simulink model "Pretty_Lin_Hover_Sim"  (R2025b)
settings: Solver=VariableStepAuto  StartTime=0.0  StopTime=10.0  RelTol=1e-3
values from neighbouring files (symbols this model uses):
  A = zeros(12,12)    [lin_hover.m]
  A_kfd = sys_kf_d.A    [lin_hover.m]
  B = zeros(12,4)    [lin_hover.m]
  B_kfd = sys_kf_d.B    [lin_hover.m]
  C11 = 4.58e-4    (= 0.000458)    [lin_hover.m]    (also in non_lin_sim.m)
  g = 9.81    [lin_hover.m]    (also in non_lin_sim.m)
  k_tau = 0.00    (= 0)    [lin_hover.m]    (also in non_lin_sim.m)
  m = 0.110    (= 0.11)    [lin_hover.m]    (also in non_lin_sim.m)
  max_pot = 1950    [lin_hover.m]
  noise_true = 1    [lin_hover.m]
  pitch_D = 0    [lin_hover.m]
  pitch_I = 0.005*Iy/Ix    [lin_hover.m]
  pitch_P = 0.022*Iy/Ix    [lin_hover.m]
  roll_D = 0    [lin_hover.m]
  roll_I = 0.005    [lin_hover.m]
  roll_P = 0.022    [lin_hover.m]
  S = 0.11    [lin_hover.m]    (also in non_lin_sim.m)
  strength = 50    [lin_hover.m]
  tau_wing = 0.1/2.2    (= 0.0454545454545)    [lin_hover.m]
  Ts = 1/fs    (= 0.00025)    [lin_hover.m]
  u0 = (m*g/4 - C21)/C11    (= 1816.10262009)    [lin_hover.m]
  X0 = zeros([12,1])    [lin_hover.m]
  Xref = zeros([12,1])    [lin_hover.m]
  Xu = rho*CDx*Ax*v_ref    (= 0.148971998855)    [lin_hover.m]    (also in non_lin_sim.m)
  yaw_D = 0    [lin_hover.m]
  yaw_I = 0.001    [lin_hover.m]
  yaw_P = 0.001    [lin_hover.m]
  Yv = rho*CDy*Ay*v_ref    (= 0.148971998855)    [lin_hover.m]    (also in non_lin_sim.m)
  Zw = rho*CDz*Az*w_ref    (= 0.104280399198)    [lin_hover.m]    (also in non_lin_sim.m)
undefined symbols (not defined in the file or in its folder): accel, C_kf, D_kf, DiscIntNeverNeededParam, Discrete, gyro, mahoney, R_kf, Time, x_kf0
libraries: slpidlib x5, simulink x3, ctrlSharedLib x1
settings Model: Creator=bmatt  LastModifiedBy=bmatt

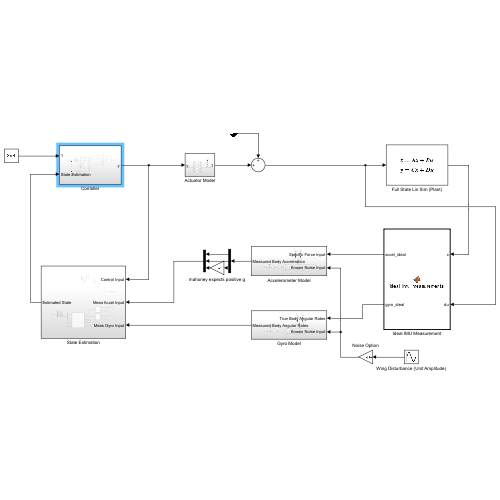
[thumbnail: Simulink's stored preview of the top-level diagram]
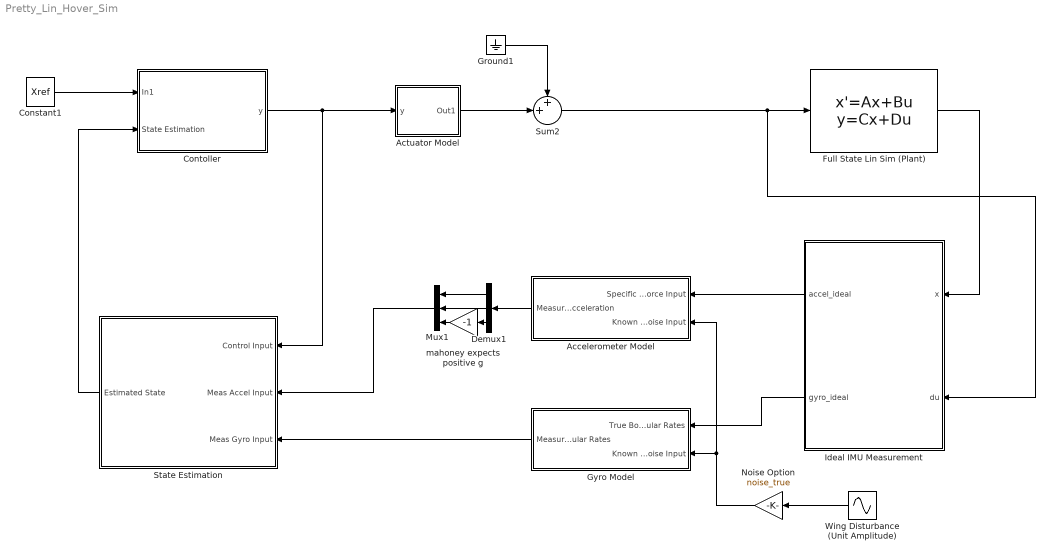
== system Pretty_Lin_Hover_Sim ==
  Accelerometer Model : Subsystem
  Actuator Model : Subsystem
  Constant1 : Constant  Value=Xref  SampleTime=-1
  Contoller : Subsystem
  Demux1 : Demux  Outputs=3
  Full State Lin Sim (Plant) : StateSpace  A=A  B=B  C=eye(12)  D=zeros(12,4)  InitialCondition=X0
  Ground1 : Ground
  Gyro Model : Subsystem
  Ideal IMU Measurement : MATLAB Function  TreatAsAtomicUnit=on
  Mux1 : Mux  Inputs=3
  Noise Option : Gain  Gain=noise_true
  State Estimation : Subsystem
  Sum2 : Sum  Inputs=++|
  Wing Disturbance (Unit Amplitude) : Sin  Frequency=2*pi*24  SampleTime=0
  mahoney expects positive g : Gain  Gain=-1
  wires:
  Sum2/1 -> Ideal IMU Measurement/2(du), Full State Lin Sim (Plant)/1
  Constant1/1 -> Contoller/1(In1)
  Actuator Model/1(Out1) -> Sum2/2
  Noise Option/1 -> Accelerometer Model/2(Known Noise Input), Gyro Model/2(Known Noise Input)
  Mux1/1 -> State Estimation/2(Meas Accel Input)
  Demux1/3 -> mahoney expects positive g/1
  State Estimation/1(Estimated State) -> Contoller/2(State Estimation)
  mahoney expects positive g/1 -> Mux1/3
  Wing Disturbance (Unit Amplitude)/1 -> Noise Option/1
  Ideal IMU Measurement/2(gyro_ideal) -> Gyro Model/1(True Body Angular Rates)
  Gyro Model/1(Measured Body Angular Rates) -> State Estimation/3(Meas Gyro Input)
  Full State Lin Sim (Plant)/1 -> Ideal IMU Measurement/1(x)
  Accelerometer Model/1(Measured Body Acceleration) -> Demux1/1
  Contoller/1(y) -> State Estimation/1(Control Input), Actuator Model/1(y)
  Demux1/1 -> Mux1/1
  Ground1/1 -> Sum2/1
  Demux1/2 -> Mux1/2
  Ideal IMU Measurement/1(accel_ideal) -> Accelerometer Model/1(Specific Force Input)

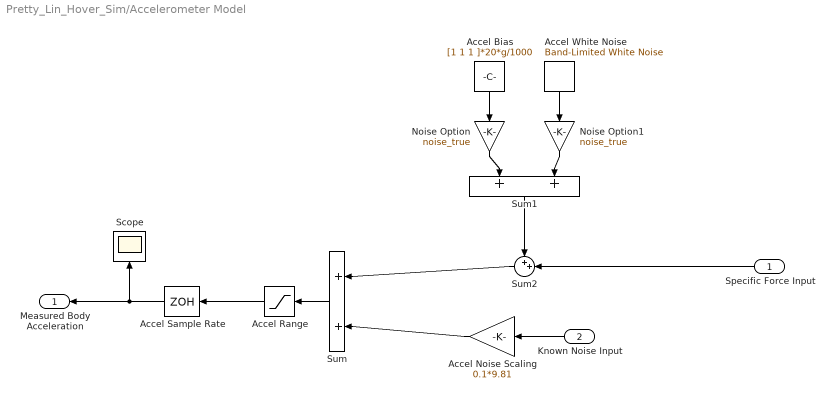
== system Pretty_Lin_Hover_Sim/Accelerometer Model ==
  Specific Force Input : Inport
  Known Noise Input : Inport  Port=2
  Accel White Noise : simulink/Sources/Band-Limited White Noise  Cov=[1 1 1]*((0.16*9.81/1000)*sqrt(740))^2  Ts=1/1600  seed=[23341]
  Accel Bias : Constant  Value=[1 1 1 ]*20*g/1000  SampleTime=1/1600
  Accel Noise Scaling : Gain  Gain=0.1*9.81
  Accel Range : Saturate  UpperLimit=4*9.81  LowerLimit=-4*9.81
  Accel Sample Rate : ZeroOrderHold  SampleTime=1/1600
  Noise Option : Gain  Gain=noise_true
  Noise Option1 : Gain  Gain=noise_true
  Scope : Scope
      settings: ActiveDisplayYMinimum=-1  ActiveDisplayYMaximum=1  DataLoggingVariableName=ScopeData13
  Sum : Sum  Inputs=+|+
  Sum1 : Sum  Inputs=+|+
  Sum2 : Sum  Inputs=++|
  Measured Body Acceleration : Outport
  wires:
  Sum/1 -> Accel Range/1
  Sum2/1 -> Sum/1
  Accel Sample Rate/1 -> Scope/1, Measured Body Acceleration/1
  Known Noise Input/1 -> Accel Noise Scaling/1
  Specific Force Input/1 -> Sum2/2
  Sum1/1 -> Sum2/1
  Accel Noise Scaling/1 -> Sum/2
  Accel Range/1 -> Accel Sample Rate/1
  Noise Option/1 -> Sum1/1
  Accel Bias/1 -> Noise Option/1
  Noise Option1/1 -> Sum1/2
  Accel White Noise/1 -> Noise Option1/1

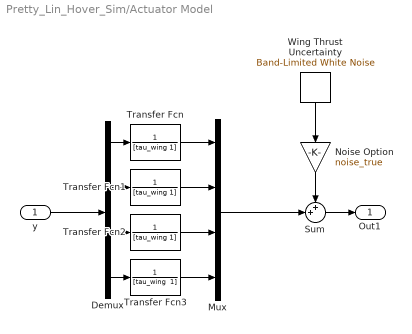
== system Pretty_Lin_Hover_Sim/Actuator Model ==
  y : Inport
  Demux : Demux
  Mux : Mux
  Noise Option : Gain  Gain=noise_true
  Sum : Sum  Inputs=++|
  Transfer Fcn : TransferFcn  Denominator=[tau_wing 1]
  Transfer Fcn1 : TransferFcn  Denominator=[tau_wing 1]
  Transfer Fcn2 : TransferFcn  Denominator=[tau_wing 1]
  Transfer Fcn3 : TransferFcn  Denominator="[tau_wing  1]"
  Wing Thrust Uncertainty : simulink/Sources/Band-Limited White Noise  Cov=1*[0.000001566122567;0.000001566122567;0.000001566122567;0.000001566122567]  Ts=Ts  seed=[23341]
  Out1 : Outport
  wires:
  Demux/4 -> Transfer Fcn3/1
  Demux/1 -> Transfer Fcn/1
  Demux/2 -> Transfer Fcn1/1
  Demux/3 -> Transfer Fcn2/1
  Transfer Fcn/1 -> Mux/1
  Transfer Fcn1/1 -> Mux/2
  Transfer Fcn2/1 -> Mux/3
  Transfer Fcn3/1 -> Mux/4
  y/1 -> Demux/1
  Sum/1 -> Out1/1
  Mux/1 -> Sum/2
  Wing Thrust Uncertainty/1 -> Noise Option/1
  Noise Option/1 -> Sum/1

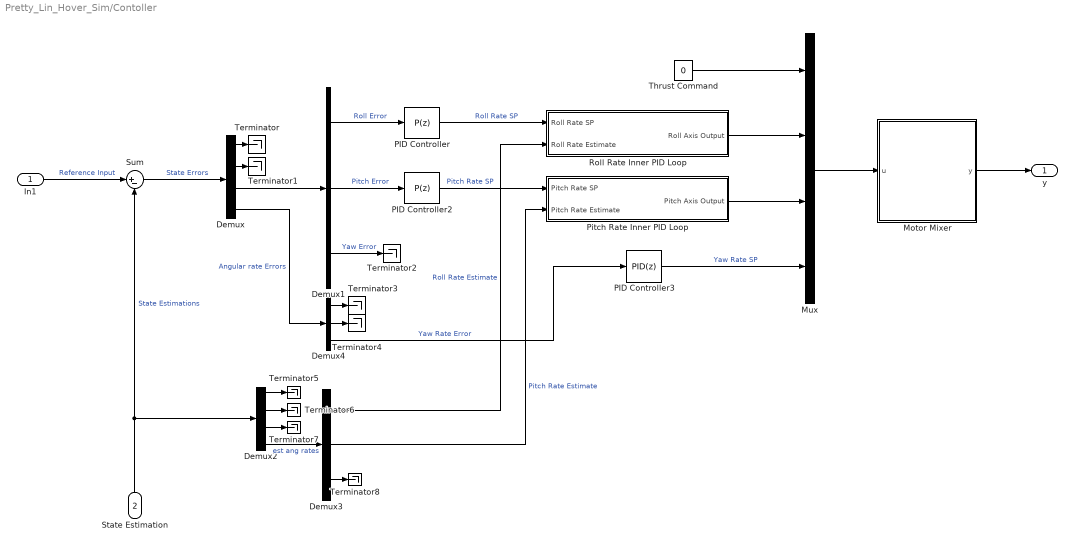
== system Pretty_Lin_Hover_Sim/Contoller ==
  In1 : Inport
  State Estimation : Inport  Port=2
  Demux : Demux  Outputs=[3 3 3 3]
  Demux1 : Demux  Outputs=[1 1 1]
  Demux2 : Demux  Outputs=[3 3 3 3]
  Demux3 : Demux  Outputs=[1 1 1]
  Demux4 : Demux  Outputs=[1 1 1]
  Motor Mixer : Subsystem
  Mux : Mux
  PID Controller : slpidlib/PID Controller  Controller=P  Form=Parallel  TimeDomain=Discrete-time  UseExternalTs=off  SampleTime=Ts  IntegratorMethod=Forward Euler  FilterMethod=Forward Euler  ControllerParametersSource=internal  P=strength/10  I=194.232873086371  UseKiTs=off  D=-0.0894221705749344  UseExternalDerivativeSource=off  N=55.5911819026225  UseFilter=on  TunerSelectOption=Frequency Response Based  InitialConditionSource=internal  InitialConditionForIntegrator=Xref(7) - X0(7)  InitialConditionForFilter=0  DifferentiatorICPrevScaledInput=0  ExternalReset=none  TrackingMode=off  Kt=1  LimitOutput=on  SatLimitsSource=internal  UpperSaturationLimit=3.5  LowerSaturationLimit=-3.5  LinearizeAsGain=on  AntiWindupMode=external  Kb=1  LimitIntegrator=off  UpperIntegratorSaturationLimit=inf  LowerIntegratorSaturationLimit=-inf  POutMin=[]  POutMax=[]  IOutMin=[]  IOutMax=[]  DOutMin=[]  DOutMax=[]  NOutMin=[]  NOutMax=[]  SumOutMin=[]  SumOutMax=[]  SaturationOutMin=[]  SaturationOutMax=[]  PParamMin=[]  PParamMax=[]  IParamMin=[]  IParamMax=[]  DParamMin=[]  DParamMax=[]  NParamMin=[]  NParamMax=[]  KbParamMin=[]  KbParamMax=[]  KtParamMin=[]  KtParamMax=[]  KbOutMin=[]  KbOutMax=[]  KtOutMin=[]  KtOutMax=[]  IntegratorOutMin=[]  IntegratorOutMax=[]  FilterOutMin=[]  FilterOutMax=[]  SumI1OutMin=[]  SumI1OutMax=[]  SumI2OutMin=[]  SumI2OutMax=[]  SumI3OutMin=[]  SumI3OutMax=[]  SumI4OutMin=[]  SumI4OutMax=[]  SumDOutMin=[]  SumDOutMax=[]  DifferentiatorOutMin=[]  DifferentiatorOutMax=[]  FilterDiffOutCoefMin=[]  FilterDiffOutCoefMax=[]  ReciprocalOutMin=[]  ReciprocalOutMax=[]  SumDenOutMin=[]  SumDenOutMax=[]  SumNumOutMin=[]  SumNumOutMax=[]  DivideOutMin=[]  DivideOutMax=[]  UdiffTsProdOutMin=[]  UdiffTsProdOutMax=[]  NTsProdOutMin=[]  NTsProdOutMax=[]  UintegralTsProdOutMin=[]  UintegralTsProdOutMax=[]  UngainTsProdOutMin=[]  UngainTsProdOutMax=[]  ClampingZeroOutDataTypeStr=Inherit: Inherit via back propagation  ClampingZeroOutMin=[]  ClampingZeroOutMax=[]  FilterDenConstantOutDataTypeStr=Inherit: Inherit via back propagation  FilterDenConstantOutMin=[]  FilterDenConstantOutMax=[]  PCopyOutDataTypeStr=Inherit: Inherit via back propagation  PCopyOutMin=[]  PCopyOutMax=[]  NCopyOutDataTypeStr=Inherit: Inherit via back propagation  NCopyOutMin=[]  NCopyOutMax=[]  IntegratorContinuousStateAttributes=''  IntegratorStateMustResolveToSignalObject=off  IntegratorRTWStateStorageClass=Auto  FilterContinuousStateAttributes=''  FilterStateMustResolveToSignalObject=off  FilterRTWStateStorageClass=Auto  ParallelPVariant=InternalParameters  IdealPVariant=Disabled  IVariant=Disabled  DVariant=Disabled  IntegratorVariant=Disabled  SatVariant=Enabled  AWVariant=Disabled  PCopyVariant=Disabled  TRVariant=Disabled  FdbkBlocksVariant=Forward  IdealPFdbkVariant=Disabled  SatFdbkVariant=Disabled  DerivativeFilterVariant=Disabled  NVariant=Disabled  NCopyVariant=Disabled_SignalSpec  FilterICVariant=Disabled  IntegratorICVariant=Disabled  ExternalResetVariant=Disabled  TRSumVariant=Passthrough  SumFdbkVariant=Disabled  SumVariant=Passthrough_P  TsampFilterVariant=InternalTs  TsampNgainVariant=Passthrough  TsampIntegralVariant=Disabled_SignalSpec  ExternalSaturationOutDataTypeStr=Inherit: Same as second input  DerivativeSourceVariant=Disabled  PreIntVariant=InternalPreInt
  PID Controller2 : slpidlib/PID Controller  Controller=P  Form=Parallel  TimeDomain=Discrete-time  UseExternalTs=off  SampleTime=Ts  IntegratorMethod=Forward Euler  FilterMethod=Forward Euler  ControllerParametersSource=internal  P=strength/10  I=0.287608182877056  UseKiTs=off  D=0  UseExternalDerivativeSource=off  N=100  UseFilter=on  TunerSelectOption=Transfer Function Based (PID Tuner App)  InitialConditionSource=internal  InitialConditionForIntegrator=Xref(8) - X0(8)  InitialConditionForFilter=0  DifferentiatorICPrevScaledInput=0  ExternalReset=none  TrackingMode=off  Kt=1  LimitOutput=on  SatLimitsSource=internal  UpperSaturationLimit=3.5  LowerSaturationLimit=-3.5  LinearizeAsGain=off  AntiWindupMode=none  Kb=1  LimitIntegrator=off  UpperIntegratorSaturationLimit=inf  LowerIntegratorSaturationLimit=-inf  POutMin=[]  POutMax=[]  IOutMin=[]  IOutMax=[]  DOutMin=[]  DOutMax=[]  NOutMin=[]  NOutMax=[]  SumOutMin=[]  SumOutMax=[]  SaturationOutMin=[]  SaturationOutMax=[]  PParamMin=[]  PParamMax=[]  IParamMin=[]  IParamMax=[]  DParamMin=[]  DParamMax=[]  NParamMin=[]  NParamMax=[]  KbParamMin=[]  KbParamMax=[]  KtParamMin=[]  KtParamMax=[]  KbOutMin=[]  KbOutMax=[]  KtOutMin=[]  KtOutMax=[]  IntegratorOutMin=[]  IntegratorOutMax=[]  FilterOutMin=[]  FilterOutMax=[]  SumI1OutMin=[]  SumI1OutMax=[]  SumI2OutMin=[]  SumI2OutMax=[]  SumI3OutMin=[]  SumI3OutMax=[]  SumI4OutMin=[]  SumI4OutMax=[]  SumDOutMin=[]  SumDOutMax=[]  DifferentiatorOutMin=[]  DifferentiatorOutMax=[]  FilterDiffOutCoefMin=[]  FilterDiffOutCoefMax=[]  ReciprocalOutMin=[]  ReciprocalOutMax=[]  SumDenOutMin=[]  SumDenOutMax=[]  SumNumOutMin=[]  SumNumOutMax=[]  DivideOutMin=[]  DivideOutMax=[]  UdiffTsProdOutMin=[]  UdiffTsProdOutMax=[]  NTsProdOutMin=[]  NTsProdOutMax=[]  UintegralTsProdOutMin=[]  UintegralTsProdOutMax=[]  UngainTsProdOutMin=[]  UngainTsProdOutMax=[]  ClampingZeroOutDataTypeStr=Inherit: Inherit via back propagation  ClampingZeroOutMin=[]  ClampingZeroOutMax=[]  FilterDenConstantOutDataTypeStr=Inherit: Inherit via back propagation  FilterDenConstantOutMin=[]  FilterDenConstantOutMax=[]  PCopyOutDataTypeStr=Inherit: Inherit via back propagation  PCopyOutMin=[]  PCopyOutMax=[]  NCopyOutDataTypeStr=Inherit: Inherit via back propagation  NCopyOutMin=[]  NCopyOutMax=[]  IntegratorContinuousStateAttributes=''  IntegratorStateMustResolveToSignalObject=off  IntegratorRTWStateStorageClass=Auto  FilterContinuousStateAttributes=''  FilterStateMustResolveToSignalObject=off  FilterRTWStateStorageClass=Auto  ParallelPVariant=InternalParameters  IdealPVariant=Disabled  IVariant=Disabled  DVariant=Disabled  IntegratorVariant=Disabled  SatVariant=Enabled  AWVariant=Disabled  PCopyVariant=Disabled  TRVariant=Disabled  FdbkBlocksVariant=Forward  IdealPFdbkVariant=Disabled  SatFdbkVariant=Disabled  DerivativeFilterVariant=Disabled  NVariant=Disabled  NCopyVariant=Disabled_SignalSpec  FilterICVariant=Disabled  IntegratorICVariant=Disabled  ExternalResetVariant=Disabled  TRSumVariant=Passthrough  SumFdbkVariant=Disabled  SumVariant=Passthrough_P  TsampFilterVariant=InternalTs  TsampNgainVariant=Passthrough  TsampIntegralVariant=Disabled_SignalSpec  ExternalSaturationOutDataTypeStr=Inherit: Same as second input  DerivativeSourceVariant=Disabled  PreIntVariant=InternalPreInt
  PID Controller3 : slpidlib/PID Controller  Controller=PID  Form=Parallel  TimeDomain=Discrete-time  UseExternalTs=off  SampleTime=Ts  IntegratorMethod=Forward Euler  FilterMethod=Forward Euler  ControllerParametersSource=internal  P=yaw_P  I=yaw_I  UseKiTs=off  D=yaw_D  UseExternalDerivativeSource=off  N=44.2614212635521  UseFilter=on  TunerSelectOption=Transfer Function Based (PID Tuner App)  InitialConditionSource=internal  InitialConditionForIntegrator=Xref(12) - X0(12)  InitialConditionForFilter=0  DifferentiatorICPrevScaledInput=0  ExternalReset=none  TrackingMode=off  Kt=1  LimitOutput=on  SatLimitsSource=internal  UpperSaturationLimit=50  LowerSaturationLimit=-50  LinearizeAsGain=on  AntiWindupMode=clamping  Kb=1  LimitIntegrator=off  UpperIntegratorSaturationLimit=inf  LowerIntegratorSaturationLimit=-inf  POutMin=[]  POutMax=[]  IOutMin=[]  IOutMax=[]  DOutMin=[]  DOutMax=[]  NOutMin=[]  NOutMax=[]  SumOutMin=[]  SumOutMax=[]  SaturationOutMin=[]  SaturationOutMax=[]  PParamMin=[]  PParamMax=[]  IParamMin=[]  IParamMax=[]  DParamMin=[]  DParamMax=[]  NParamMin=[]  NParamMax=[]  KbParamMin=[]  KbParamMax=[]  KtParamMin=[]  KtParamMax=[]  KbOutMin=[]  KbOutMax=[]  KtOutMin=[]  KtOutMax=[]  IntegratorOutMin=[]  IntegratorOutMax=[]  FilterOutMin=[]  FilterOutMax=[]  SumI1OutMin=[]  SumI1OutMax=[]  SumI2OutMin=[]  SumI2OutMax=[]  SumI3OutMin=[]  SumI3OutMax=[]  SumI4OutMin=[]  SumI4OutMax=[]  SumDOutMin=[]  SumDOutMax=[]  DifferentiatorOutMin=[]  DifferentiatorOutMax=[]  FilterDiffOutCoefMin=[]  FilterDiffOutCoefMax=[]  ReciprocalOutMin=[]  ReciprocalOutMax=[]  SumDenOutMin=[]  SumDenOutMax=[]  SumNumOutMin=[]  SumNumOutMax=[]  DivideOutMin=[]  DivideOutMax=[]  UdiffTsProdOutMin=[]  UdiffTsProdOutMax=[]  NTsProdOutMin=[]  NTsProdOutMax=[]  UintegralTsProdOutMin=[]  UintegralTsProdOutMax=[]  UngainTsProdOutMin=[]  UngainTsProdOutMax=[]  ClampingZeroOutDataTypeStr=Inherit: Inherit via back propagation  ClampingZeroOutMin=[]  ClampingZeroOutMax=[]  FilterDenConstantOutDataTypeStr=Inherit: Inherit via back propagation  FilterDenConstantOutMin=[]  FilterDenConstantOutMax=[]  PCopyOutDataTypeStr=Inherit: Inherit via back propagation  PCopyOutMin=[]  PCopyOutMax=[]  NCopyOutDataTypeStr=Inherit: Inherit via back propagation  NCopyOutMin=[]  NCopyOutMax=[]  IntegratorContinuousStateAttributes=''  IntegratorStateMustResolveToSignalObject=off  IntegratorRTWStateStorageClass=Auto  FilterContinuousStateAttributes=''  FilterStateMustResolveToSignalObject=off  FilterRTWStateStorageClass=Auto  ParallelPVariant=InternalParameters  IdealPVariant=Disabled  IVariant=InternalParameters  DVariant=InternalParameters  IntegratorVariant=Discrete  SatVariant=Enabled  AWVariant=DiscClampingParallel  PCopyVariant=Disabled  TRVariant=Disabled  FdbkBlocksVariant=Forward  IdealPFdbkVariant=Disabled  SatFdbkVariant=Disabled  DerivativeFilterVariant=ForwardEulerFilter  NVariant=InternalParameters  NCopyVariant=Disabled  FilterICVariant=InternalICsFilter  IntegratorICVariant=InternalICs  ExternalResetVariant=Disabled  TRSumVariant=Passthrough  SumFdbkVariant=Disabled  SumVariant=Sum_PID  TsampFilterVariant=InternalTs  TsampNgainVariant=Passthrough  TsampIntegralVariant=Disabled_SignalSpec  ExternalSaturationOutDataTypeStr=Inherit: Same as second input  DerivativeSourceVariant=ErrorSignal  PreIntVariant=InternalPreInt
  Pitch Rate Inner PID Loop : Subsystem
  Roll Rate Inner PID Loop : Subsystem
  Sum : Sum  Inputs=|+-
  Terminator{,1..8} (9 alike) : Terminator
  Thrust Command : Constant  Value=0
  y : Outport
  wires:
  In1/1 -> Sum/1  "Reference Input"
  State Estimation/1 -> Demux2/1, Sum/2  "State Estimations"
  Sum/1 -> Demux/1  "State Errors"
  Demux/3 -> Demux1/1
  Demux2/4 -> Demux3/1  "est ang rates"
  Demux1/2 -> PID Controller2/1  "Pitch Error"
  Demux3/1 -> Roll Rate Inner PID Loop/2(Roll Rate Estimate)  "Roll Rate Estimate"
  PID Controller2/1 -> Pitch Rate Inner PID Loop/1(Pitch Rate SP)  "Pitch Rate SP"
  Demux3/2 -> Pitch Rate Inner PID Loop/2(Pitch Rate Estimate)  "Pitch Rate Estimate"
  Demux/4 -> Demux4/1  "Angular rate Errors"
  Demux4/3 -> PID Controller3/1  "Yaw Rate Error"
  Roll Rate Inner PID Loop/1(Roll Axis Output) -> Mux/2
  Pitch Rate Inner PID Loop/1(Pitch Axis Output) -> Mux/3
  PID Controller3/1 -> Mux/4  "Yaw Rate SP"
  Demux/1 -> Terminator/1
  Demux/2 -> Terminator1/1
  Demux1/3 -> Terminator2/1  "Yaw Error"
  Demux4/1 -> Terminator3/1
  Demux4/2 -> Terminator4/1
  Demux2/1 -> Terminator5/1
  Demux2/2 -> Terminator6/1
  Demux2/3 -> Terminator7/1
  Demux3/3 -> Terminator8/1
  Demux1/1 -> PID Controller/1  "Roll Error"
  Thrust Command/1 -> Mux/1
  PID Controller/1 -> Roll Rate Inner PID Loop/1(Roll Rate SP)  "Roll Rate SP"
  Mux/1 -> Motor Mixer/1(u)
  Motor Mixer/1(y) -> y/1

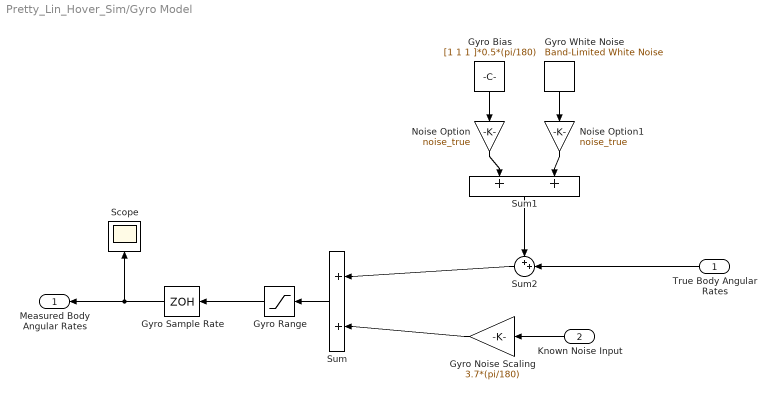
== system Pretty_Lin_Hover_Sim/Gyro Model ==
  True Body Angular Rates : Inport
  Known Noise Input : Inport  Port=2
  Gyro White Noise : simulink/Sources/Band-Limited White Noise  Cov=[1 1 1]*(0.007*(pi/180)*sqrt(751))^2  Ts=1/3200  seed=[23341]
  Gyro Bias : Constant  Value=[1 1 1 ]*0.5*(pi/180)  SampleTime=1/3200
  Gyro Noise Scaling : Gain  Gain=3.7*(pi/180)
  Gyro Range : Saturate  UpperLimit=1000*(pi/180)  LowerLimit=-1000*(pi/180)
  Gyro Sample Rate : ZeroOrderHold  SampleTime=1/3200
  Noise Option : Gain  Gain=noise_true
  Noise Option1 : Gain  Gain=noise_true
  Scope : Scope
      settings: ActiveDisplayYMinimum=-1  ActiveDisplayYMaximum=1  DataLoggingVariableName=ScopeData14
  Sum : Sum  Inputs=+|+
  Sum1 : Sum  Inputs=+|+
  Sum2 : Sum  Inputs=++|
  Measured Body Angular Rates : Outport
  wires:
  Sum/1 -> Gyro Range/1
  Known Noise Input/1 -> Gyro Noise Scaling/1
  Sum1/1 -> Sum2/1
  True Body Angular Rates/1 -> Sum2/2
  Gyro Sample Rate/1 -> Scope/1, Measured Body Angular Rates/1
  Gyro Range/1 -> Gyro Sample Rate/1
  Sum2/1 -> Sum/1
  Gyro Noise Scaling/1 -> Sum/2
  Noise Option/1 -> Sum1/1
  Gyro Bias/1 -> Noise Option/1
  Gyro White Noise/1 -> Noise Option1/1
  Noise Option1/1 -> Sum1/2

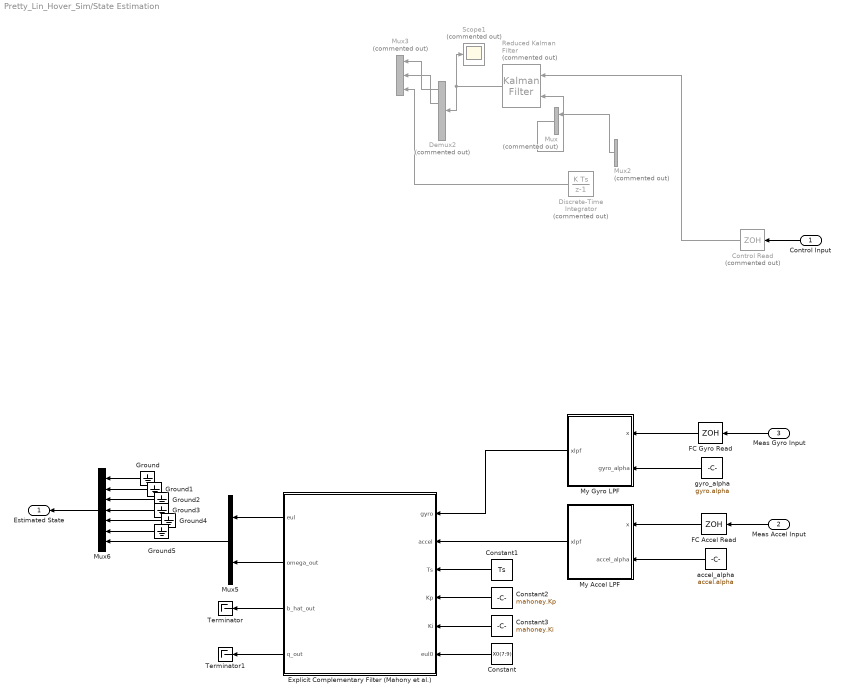
== system Pretty_Lin_Hover_Sim/State Estimation ==
  Control Input : Inport
  Meas Accel Input : Inport  Port=2
  Meas Gyro Input : Inport  Port=3
  Constant : Constant  Value=X0(7:9)
  Constant1 : Constant  Value=Ts
  Constant2 : Constant  Value=mahoney.Kp
  Constant3 : Constant  Value=mahoney.Ki
  Control Read : ZeroOrderHold  Commented=on  SampleTime=Ts
  Demux2 : Demux  Commented=on  Outputs=[1 1 1 1]
  Discrete-Time Integrator : DiscreteIntegrator  Commented=on  InitialCondition=X0(9)  SampleTime=-1  ICPrevOutput=DiscIntNeverNeededParam  ICPrevScaledInput=DiscIntNeverNeededParam
  Explicit Complementary Filter (Mahony et al.) : MATLAB Function  TreatAsAtomicUnit=on
  FC Accel Read : ZeroOrderHold  SampleTime=Ts
  FC Gyro Read : ZeroOrderHold  SampleTime=Ts
  Ground{,1..5} (6 alike) : Ground
  Mux : Mux  Commented=on  Inputs=2
  Mux2 : Mux  Commented=on  Inputs=2
  Mux3 : Mux  Commented=on  Inputs=3
  Mux5 : Mux  Inputs=2
  Mux6 : Mux  Inputs=7
  My Accel LPF : MATLAB Function  TreatAsAtomicUnit=on
  My Gyro LPF : MATLAB Function  TreatAsAtomicUnit=on
  Reduced Kalman Filter : ctrlSharedLib/Kalman Filter  Commented=on  TimeDomain=Discrete-Time  UseCurrentEstimator=on  ModelSource=Individual A, B, C, D matrices  ModelSourceVariable=ss(0.95,1,1,0,1)  A=A_kfd  B=B_kfd  C=C_kf  D=D_kf  NumberOfStates=1  NumberOfInputs=1  NumberOfOutputs=1  InitialEstimateSource=Dialog  X0=x_kf0  P0=10  UseK=off  UseGH=off  NumberOfProcessNoiseInputs=1  G=1  TimeInvariantG=on  H=0  TimeInvariantH=on  Q=Q_kf  TimeInvariantQ=on  R=R_kf  TimeInvariantR=on  N=0  TimeInvariantN=on  AddInputPort=on  AddEnablePort=off  OutputEstimatedY=off  OutputP=off  Ts=Ts
  Scope1 : Scope  Commented=on
      settings: ActiveDisplayYMinimum=-1.3309196424589129  ActiveDisplayYMaximum=1.1359717359097128  DataLoggingVariableName=ScopeData12
  Terminator : Terminator
  Terminator1 : Terminator
  accel_alpha : Constant  Value=accel.alpha
  gyro_alpha : Constant  Value=gyro.alpha
  Estimated State : Outport
  wires:
  Meas Gyro Input/1 -> FC Gyro Read/1
  Meas Accel Input/1 -> FC Accel Read/1
  Mux/1 -> Reduced Kalman Filter/2
  Control Input/1 -> Control Read/1
  FC Gyro Read/1 -> My Gyro LPF/1(x)
  Reduced Kalman Filter/1 -> Demux2/1, Scope1/1
  Demux2/1 -> Mux3/1
  Demux2/2 -> Mux3/2
  Mux5/1 -> Mux6/7
  Control Read/1 -> Reduced Kalman Filter/1
  Mux2/1 -> Mux/1
  Mux6/1 -> Estimated State/1
  Ground/1 -> Mux6/1
  Ground1/1 -> Mux6/2
  Ground2/1 -> Mux6/3
  Ground3/1 -> Mux6/4
  Ground4/1 -> Mux6/5
  Ground5/1 -> Mux6/6
  My Gyro LPF/1(xlpf) -> Explicit Complementary Filter (Mahony et al.)/1(gyro)
  gyro_alpha/1 -> My Gyro LPF/2(gyro_alpha)
  FC Accel Read/1 -> My Accel LPF/1(x)
  My Accel LPF/1(xlpf) -> Explicit Complementary Filter (Mahony et al.)/2(accel)
  Explicit Complementary Filter (Mahony et al.)/1(eul) -> Mux5/1
  Discrete-Time Integrator/1 -> Mux3/3
  Constant1/1 -> Explicit Complementary Filter (Mahony et al.)/3(Ts)
  accel_alpha/1 -> My Accel LPF/2(accel_alpha)
  Constant/1 -> Explicit Complementary Filter (Mahony et al.)/6(eul0)
  Constant2/1 -> Explicit Complementary Filter (Mahony et al.)/4(Kp)
  Constant3/1 -> Explicit Complementary Filter (Mahony et al.)/5(Ki)
  Explicit Complementary Filter (Mahony et al.)/3(b_hat_out) -> Terminator/1
  Explicit Complementary Filter (Mahony et al.)/4(q_out) -> Terminator1/1
  Explicit Complementary Filter (Mahony et al.)/2(omega_out) -> Mux5/2

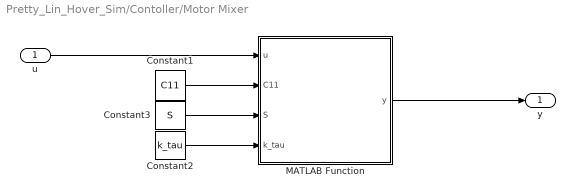
== system Pretty_Lin_Hover_Sim/Contoller/Motor Mixer ==
  u : Inport
  Constant1 : Constant  Value=C11
  Constant2 : Constant  Value=k_tau
  Constant3 : Constant  Value=S
  MATLAB Function : MATLAB Function  TreatAsAtomicUnit=on
  y : Outport
  wires:
  u/1 -> MATLAB Function/1(u)
  Constant3/1 -> MATLAB Function/3(S)
  MATLAB Function/1(y) -> y/1
  Constant2/1 -> MATLAB Function/4(k_tau)
  Constant1/1 -> MATLAB Function/2(C11)

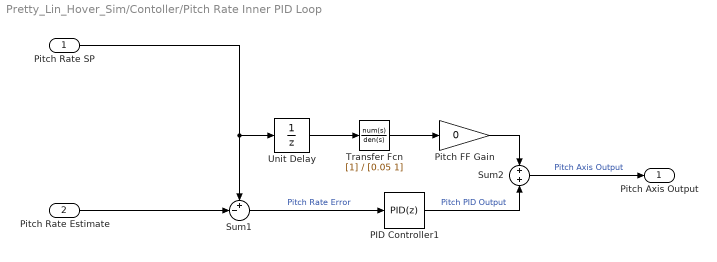
== system Pretty_Lin_Hover_Sim/Contoller/Pitch Rate Inner PID Loop ==
  Pitch Rate SP : Inport
  Pitch Rate Estimate : Inport  Port=2
  PID Controller1 : slpidlib/PID Controller  Controller=PID  Form=Parallel  TimeDomain=Discrete-time  UseExternalTs=off  SampleTime=Ts  IntegratorMethod=Forward Euler  FilterMethod=Forward Euler  ControllerParametersSource=internal  P=pitch_P  I=pitch_I  UseKiTs=off  D=pitch_D  UseExternalDerivativeSource=off  N=40  UseFilter=on  TunerSelectOption=Transfer Function Based (PID Tuner App)  InitialConditionSource=internal  InitialConditionForIntegrator=Xref(11) - X0(11)  InitialConditionForFilter=0  DifferentiatorICPrevScaledInput=0  ExternalReset=none  TrackingMode=off  Kt=1  LimitOutput=on  SatLimitsSource=internal  UpperSaturationLimit=S*C11*(2*(max_pot-u0))  LowerSaturationLimit=-S*C11*(2*(max_pot-u0))  LinearizeAsGain=on  AntiWindupMode=clamping  Kb=1  LimitIntegrator=off  UpperIntegratorSaturationLimit=inf  LowerIntegratorSaturationLimit=-inf  POutMin=[]  POutMax=[]  IOutMin=[]  IOutMax=[]  DOutMin=[]  DOutMax=[]  NOutMin=[]  NOutMax=[]  SumOutMin=[]  SumOutMax=[]  SaturationOutMin=[]  SaturationOutMax=[]  PParamMin=[]  PParamMax=[]  IParamMin=[]  IParamMax=[]  DParamMin=[]  DParamMax=[]  NParamMin=[]  NParamMax=[]  KbParamMin=[]  KbParamMax=[]  KtParamMin=[]  KtParamMax=[]  KbOutMin=[]  KbOutMax=[]  KtOutMin=[]  KtOutMax=[]  IntegratorOutMin=[]  IntegratorOutMax=[]  FilterOutMin=[]  FilterOutMax=[]  SumI1OutMin=[]  SumI1OutMax=[]  SumI2OutMin=[]  SumI2OutMax=[]  SumI3OutMin=[]  SumI3OutMax=[]  SumI4OutMin=[]  SumI4OutMax=[]  SumDOutMin=[]  SumDOutMax=[]  DifferentiatorOutMin=[]  DifferentiatorOutMax=[]  FilterDiffOutCoefMin=[]  FilterDiffOutCoefMax=[]  ReciprocalOutMin=[]  ReciprocalOutMax=[]  SumDenOutMin=[]  SumDenOutMax=[]  SumNumOutMin=[]  SumNumOutMax=[]  DivideOutMin=[]  DivideOutMax=[]  UdiffTsProdOutMin=[]  UdiffTsProdOutMax=[]  NTsProdOutMin=[]  NTsProdOutMax=[]  UintegralTsProdOutMin=[]  UintegralTsProdOutMax=[]  UngainTsProdOutMin=[]  UngainTsProdOutMax=[]  ClampingZeroOutDataTypeStr=Inherit: Inherit via back propagation  ClampingZeroOutMin=[]  ClampingZeroOutMax=[]  FilterDenConstantOutDataTypeStr=Inherit: Inherit via back propagation  FilterDenConstantOutMin=[]  FilterDenConstantOutMax=[]  PCopyOutDataTypeStr=Inherit: Inherit via back propagation  PCopyOutMin=[]  PCopyOutMax=[]  NCopyOutDataTypeStr=Inherit: Inherit via back propagation  NCopyOutMin=[]  NCopyOutMax=[]  IntegratorContinuousStateAttributes=''  IntegratorStateMustResolveToSignalObject=off  IntegratorRTWStateStorageClass=Auto  FilterContinuousStateAttributes=''  FilterStateMustResolveToSignalObject=off  FilterRTWStateStorageClass=Auto  ParallelPVariant=InternalParameters  IdealPVariant=Disabled  IVariant=InternalParameters  DVariant=InternalParameters  IntegratorVariant=Discrete  SatVariant=Enabled  AWVariant=DiscClampingParallel  PCopyVariant=Disabled  TRVariant=Disabled  FdbkBlocksVariant=Forward  IdealPFdbkVariant=Disabled  SatFdbkVariant=Disabled  DerivativeFilterVariant=ForwardEulerFilter  NVariant=InternalParameters  NCopyVariant=Disabled  FilterICVariant=InternalICsFilter  IntegratorICVariant=InternalICs  ExternalResetVariant=Disabled  TRSumVariant=Passthrough  SumFdbkVariant=Disabled  SumVariant=Sum_PID  TsampFilterVariant=InternalTs  TsampNgainVariant=Passthrough  TsampIntegralVariant=Disabled_SignalSpec  ExternalSaturationOutDataTypeStr=Inherit: Same as second input  DerivativeSourceVariant=ErrorSignal  PreIntVariant=InternalPreInt
  Pitch FF Gain : Gain  Gain=0
  Sum1 : Sum  Inputs=+-|
  Sum2 : Sum  Inputs=+|+
  Transfer Fcn : TransferFcn  Denominator=[0.05 1]
  Unit Delay : UnitDelay  InitialCondition=X0(8)  SampleTime=-1  HasFrameUpgradeWarning=on
  Pitch Axis Output : Outport
  wires:
  Pitch FF Gain/1 -> Sum2/1
  Pitch Rate Estimate/1 -> Sum1/2
  Transfer Fcn/1 -> Pitch FF Gain/1
  Sum2/1 -> Pitch Axis Output/1  "Pitch Axis Output"
  Pitch Rate SP/1 -> Unit Delay/1, Sum1/1
  Unit Delay/1 -> Transfer Fcn/1
  PID Controller1/1 -> Sum2/2  "Pitch PID Output"
  Sum1/1 -> PID Controller1/1  "Pitch Rate Error"

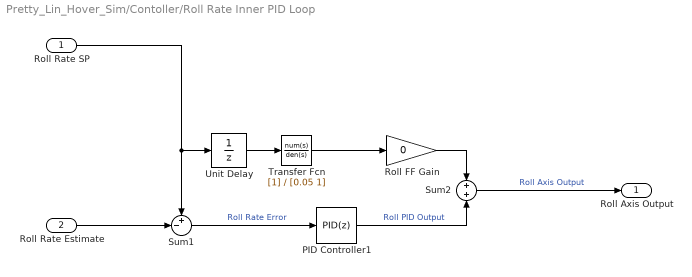
== system Pretty_Lin_Hover_Sim/Contoller/Roll Rate Inner PID Loop ==
  Roll Rate SP : Inport
  Roll Rate Estimate : Inport  Port=2
  PID Controller1 : slpidlib/PID Controller  Controller=PID  Form=Parallel  TimeDomain=Discrete-time  UseExternalTs=off  SampleTime=Ts  IntegratorMethod=Forward Euler  FilterMethod=Forward Euler  ControllerParametersSource=internal  P=roll_P  I=roll_I  UseKiTs=off  D=roll_D  UseExternalDerivativeSource=off  N=40  UseFilter=on  TunerSelectOption=Transfer Function Based (PID Tuner App)  InitialConditionSource=internal  InitialConditionForIntegrator=Xref(10) - X0(10)  InitialConditionForFilter=0  DifferentiatorICPrevScaledInput=0  ExternalReset=none  TrackingMode=off  Kt=1  LimitOutput=on  SatLimitsSource=internal  UpperSaturationLimit=S*C11*(2*(max_pot-u0))  LowerSaturationLimit=-S*C11*(2*(max_pot-u0))  LinearizeAsGain=on  AntiWindupMode=clamping  Kb=1  LimitIntegrator=off  UpperIntegratorSaturationLimit=inf  LowerIntegratorSaturationLimit=-inf  POutMin=[]  POutMax=[]  IOutMin=[]  IOutMax=[]  DOutMin=[]  DOutMax=[]  NOutMin=[]  NOutMax=[]  SumOutMin=[]  SumOutMax=[]  SaturationOutMin=[]  SaturationOutMax=[]  PParamMin=[]  PParamMax=[]  IParamMin=[]  IParamMax=[]  DParamMin=[]  DParamMax=[]  NParamMin=[]  NParamMax=[]  KbParamMin=[]  KbParamMax=[]  KtParamMin=[]  KtParamMax=[]  KbOutMin=[]  KbOutMax=[]  KtOutMin=[]  KtOutMax=[]  IntegratorOutMin=[]  IntegratorOutMax=[]  FilterOutMin=[]  FilterOutMax=[]  SumI1OutMin=[]  SumI1OutMax=[]  SumI2OutMin=[]  SumI2OutMax=[]  SumI3OutMin=[]  SumI3OutMax=[]  SumI4OutMin=[]  SumI4OutMax=[]  SumDOutMin=[]  SumDOutMax=[]  DifferentiatorOutMin=[]  DifferentiatorOutMax=[]  FilterDiffOutCoefMin=[]  FilterDiffOutCoefMax=[]  ReciprocalOutMin=[]  ReciprocalOutMax=[]  SumDenOutMin=[]  SumDenOutMax=[]  SumNumOutMin=[]  SumNumOutMax=[]  DivideOutMin=[]  DivideOutMax=[]  UdiffTsProdOutMin=[]  UdiffTsProdOutMax=[]  NTsProdOutMin=[]  NTsProdOutMax=[]  UintegralTsProdOutMin=[]  UintegralTsProdOutMax=[]  UngainTsProdOutMin=[]  UngainTsProdOutMax=[]  ClampingZeroOutDataTypeStr=Inherit: Inherit via back propagation  ClampingZeroOutMin=[]  ClampingZeroOutMax=[]  FilterDenConstantOutDataTypeStr=Inherit: Inherit via back propagation  FilterDenConstantOutMin=[]  FilterDenConstantOutMax=[]  PCopyOutDataTypeStr=Inherit: Inherit via back propagation  PCopyOutMin=[]  PCopyOutMax=[]  NCopyOutDataTypeStr=Inherit: Inherit via back propagation  NCopyOutMin=[]  NCopyOutMax=[]  IntegratorContinuousStateAttributes=''  IntegratorStateMustResolveToSignalObject=off  IntegratorRTWStateStorageClass=Auto  FilterContinuousStateAttributes=''  FilterStateMustResolveToSignalObject=off  FilterRTWStateStorageClass=Auto  ParallelPVariant=InternalParameters  IdealPVariant=Disabled  IVariant=InternalParameters  DVariant=InternalParameters  IntegratorVariant=Discrete  SatVariant=Enabled  AWVariant=DiscClampingParallel  PCopyVariant=Disabled  TRVariant=Disabled  FdbkBlocksVariant=Forward  IdealPFdbkVariant=Disabled  SatFdbkVariant=Disabled  DerivativeFilterVariant=ForwardEulerFilter  NVariant=InternalParameters  NCopyVariant=Disabled  FilterICVariant=InternalICsFilter  IntegratorICVariant=InternalICs  ExternalResetVariant=Disabled  TRSumVariant=Passthrough  SumFdbkVariant=Disabled  SumVariant=Sum_PID  TsampFilterVariant=InternalTs  TsampNgainVariant=Passthrough  TsampIntegralVariant=Disabled_SignalSpec  ExternalSaturationOutDataTypeStr=Inherit: Same as second input  DerivativeSourceVariant=ErrorSignal  PreIntVariant=InternalPreInt
  Roll FF Gain : Gain  Gain=0
  Sum1 : Sum  Inputs=+-|
  Sum2 : Sum  Inputs=+|+
  Transfer Fcn : TransferFcn  Denominator=[0.05 1]
  Unit Delay : UnitDelay  InitialCondition=X0(7)  SampleTime=-1  HasFrameUpgradeWarning=on
  Roll Axis Output : Outport
  wires:
  Roll FF Gain/1 -> Sum2/1
  Roll Rate Estimate/1 -> Sum1/2
  Transfer Fcn/1 -> Roll FF Gain/1
  PID Controller1/1 -> Sum2/2  "Roll PID Output"
  Sum1/1 -> PID Controller1/1  "Roll Rate Error"
  Unit Delay/1 -> Transfer Fcn/1
  Roll Rate SP/1 -> Unit Delay/1, Sum1/1
  Sum2/1 -> Roll Axis Output/1  "Roll Axis Output"

== matlab function Pretty_Lin_Hover_Sim/Contoller/Motor Mixer/MATLAB Function ==
  data: u input; y output; C11 input; S input; k_tau input
function y = mix_quadflapper(u, C11, S, k_tau)
% du = [du1; du2; du3; du4] consistent with your B matrix:
% B6  ~ -(C11/m) * [1 1 1 1]
% B10 ~ (S*C11/Ix) * [0 -1 0 1]
% B11 ~ (S*C11/Iy) * [1 0 -1 0]
% B12 ~ (k_tau/Iz) * [1 -1 1 -1]
    if any(~isfinite(u))
    error('Mixer input contains NaN/Inf');
    end
    % Collective per-motor increment (note sign per your B row 6)
    uT = -u(1)/(4*(C11));

    % Roll and pitch differential components
    uR = u(2)/(2*S*C11);   % makes (du4 - du2) = taux/(S*C11)
    uP = u(3)/(2*S*C11);   % makes (du1 - du3) = tauy/(S*C11)

    % Yaw component (if available)
    if abs(k_tau) < 1e-12
        uY = 0;  % no yaw authority modeled
    else
        uY = u(4)/(4*k_tau); % makes (du1 - du2 + du3 - du4) = tauz/k_tau
    end
    
    
    du1 = uT + uP + uY;
    du2 = uT - uR - uY;
    du3 = uT - uP + uY;
    du4 = uT + uR - uY;

    y = [du1; du2; du3; du4];

    
end

== matlab function Pretty_Lin_Hover_Sim/Ideal IMU Measurement ==
  data: x input; accel_ideal output; du input; gyro_ideal output; m parameter; g parameter; C11 parameter; Xu parameter; Yv parameter; Zw parameter; noise_true parameter
function [accel_ideal, gyro_ideal] = ideal_imu_measurements( ...
    x, du, m, g, C11, Xu, Yv, Zw, noise_true)
%#codegen
%
% x  = [x y z u v w phi theta psi p q r]'
% du = [du1 du2 du3 du4]' motor/flapper increments from hover trim
%
% Body/NED convention:
%   body x forward
%   body y right
%   body z down
%   thrust acts in negative body-z
%
% Output:
%   accel_ideal = ideal accelerometer specific force [m/s^2]
%                 level stationary hover -> [0; 0; -g]
%   gyro_ideal  = ideal gyro measurement [rad/s]

% -----------------------------
% Extract states
% -----------------------------
u_b = x(4);
v_b = x(5);
w_b = x(6);

phi   = x(7);   % roll
theta = x(8);   % pitch
% psi not needed for gravity projection into body z-down accel convention

p = x(10);
q = x(11);
r = x(12);

% -----------------------------
% Nonlinear gravity / specific-force direction
% -----------------------------
% Ideal accelerometer at rest measures specific force opposite gravity.
%
% For body z down:
%   level stationary hover -> [0; 0; -g]
%
% Nonlinear version:
accel_gravity = [ g*sin(theta);
                 -g*sin(phi)*cos(theta);
                 -g*cos(phi)*cos(theta)];

% -----------------------------
% Simple external acceleration terms
% -----------------------------

% Linear drag/damping accelerations from your plant model
a_drag = [-(Xu/m)*u_b;
          -(Yv/m)*v_b;
          -(Zw/m)*w_b];

% Incremental thrust acceleration from your B matrix
% Since hover thrust is already represented by accel_gravity = [0;0;-g]
% only add incremental thrust from du here.
a_thrust = [0;
            0;
           -(C11/m)*sum(du)];

% -----------------------------
% Ideal accel and gyro outputs
% -----------------------------
accel_ideal = accel_gravity + noise_true*a_drag + noise_true*a_thrust;

gyro_ideal = [p;
              q;
              r];

end

== matlab function Pretty_Lin_Hover_Sim/State Estimation/Explicit Complementary Filter (Mahony et al.) ==
  data: gyro input; eul output; omega_out output; accel input; Ts input; Kp input; Ki input; eul0 input; b_hat_out output; q_out output
function [eul, omega_out, b_hat_out, q_out] = mahony_explicit_accel_only_simulink(gyro, accel, Ts, Kp, Ki, eul0)
%#codegen
% mahony_explicit_accel_only_simulink
%
% Simulink MATLAB Function block version of Mahony explicit complementary
% filter using gyro + accelerometer only.
%
% Inputs:
%   gyro  = [p; q; r] body rates in rad/s
%   accel = [ax; ay; az] accelerometer measurement
%   Ts    = sample time [s]
%   Kp    = proportional correction gain
%   Ki    = integral/bias correction gain
%   eul0  = [roll0; pitch0; yaw0] initial attitude in radians
%   reset = reset/reinitialize flag, boolean or 0/1
%
% Outputs:
%   eul       = [roll; pitch; yaw] in radians
%   b_hat_out = estimated gyro bias [rad/s]
%   q_out     = current quaternion [qw; qx; qy; qz]
%
% Notes:
%   - Roll and pitch are corrected using accelerometer.
%   - Yaw is only gyro-integrated and will drift with accel-only correction.
%   - This assumes level stationary accel is approximately [0; 0; +g].
%   - Quaternion convention is [qw; qx; qy; qz].

persistent q b_hat initialized

if isempty(initialized)
    q = eul321_to_quat(eul0(1), eul0(2), eul0(3));
    b_hat = zeros(3,1);
    initialized = true;
end

% if reset ~= 0
%     q = eul321_to_quat(eul0(1), eul0(2), eul0(3));
%     b_hat = zeros(3,1);
%     reset = 0;          % make reset false after initialization
% end

% -----------------------------
% Measurement correction
% -----------------------------
omega_mes = zeros(3,1);

accNorm = sqrt(accel(1)^2 + accel(2)^2 + accel(3)^2);

if accNorm > 1e-9

    % Measured gravity direction in body frame
    v = accel / accNorm;

    qw = q(1);
    qx = q(2);
    qy = q(3);
    qz = q(4);

    % Estimated gravity direction in body frame from current attitude
    %
    % This assumes level stationary accel is approximately [0; 0; +g].
    v_hat = [ ...
        2.0*(qx*qz - qw*qy);
        2.0*(qw*qx + qy*qz);
        qw*qw - qx*qx - qy*qy + qz*qz ];

    % Mahony explicit complementary filter innovation
    omega_mes = cross3(v, v_hat);

    % If your attitude correction diverges instead of converging,
    % flip the sign by using this instead:
    % omega_mes = cross3(v_hat, v);

end

% -----------------------------
% Bias estimate update
% -----------------------------
% This estimates gyro bias in observable directions.
% With accel-only correction, yaw bias is not observable.
b_hat = b_hat - Ki * omega_mes * Ts;

% Corrected gyro
omega = gyro - b_hat + Kp * omega_mes;

%Output Corrected rates !!!!!!!!!!!!!!!!!!!!!!!!!!!!!!!!!!!!!!!!!!!!!!!!
omega_out = gyro - b_hat; % These are the corrected body angular rates that can be used for rate control outside of this estimator

% -----------------------------
% Quaternion propagation using corrected omega
% -----------------------------
qw = q(1);
qx = q(2);
qy = q(3);
qz = q(4);

p = omega(1);
qrate = omega(2);
r = omega(3);

qdot = 0.5 * [ ...
    -qx*p - qy*qrate - qz*r;
     qw*p + qy*r     - qz*qrate;
     qw*qrate - qx*r + qz*p;
     qw*r + qx*qrate - qy*p ];

q = q + qdot * Ts;

% Normalize quaternion
qnorm = sqrt(q(1)^2 + q(2)^2 + q(3)^2 + q(4)^2);

if qnorm > 1e-12
    q = q / qnorm;
else
    q = eul321_to_quat(eul0(1), eul0(2), eul0(3));
    b_hat = zeros(3,1);
end

% -----------------------------
% Quaternion to Euler angles
% -----------------------------
qw = q(1);
qx = q(2);
qy = q(3);
qz = q(4);

roll = atan2( ...
    2.0*(qw*qx + qy*qz), ...
    1.0 - 2.0*(qx*qx + qy*qy) );

sinPitch = 2.0*(qw*qy - qz*qx);

if sinPitch > 1.0
    sinPitch = 1.0;
elseif sinPitch < -1.0
    sinPitch = -1.0;
end

pitch = asin(sinPitch);

yaw = atan2( ...
    2.0*(qw*qz + qx*qy), ...
    1.0 - 2.0*(qy*qy + qz*qz) );

% Output Euler Angles !!!!!!!!!!!!!!!!!!!!!!!!!!!!!!!!!!!!!!!!!!!!!!!!
eul = [roll; pitch; yaw];

% Output Bias Estimate and Quaternion Estimate !!!!!!!!!!!!!!!!!!!!!!!!!!!!!!!!!!!!!!!!!!!!!!!!
b_hat_out = b_hat;
q_out = q;

end


function q = eul321_to_quat(roll, pitch, yaw)
% eul321_to_quat
%
% Converts 3-2-1 yaw-pitch-roll Euler angles to quaternion [qw; qx; qy; qz].
%
% roll  = phi
% pitch = theta
% yaw   = psi

cr = cos(0.5*roll);
sr = sin(0.5*roll);

cp = cos(0.5*pitch);
sp = sin(0.5*pitch);

cy = cos(0.5*yaw);
sy = sin(0.5*yaw);

qw = cy*cp*cr + sy*sp*sr;
qx = cy*cp*sr - sy*sp*cr;
qy = cy*sp*cr + sy*cp*sr;
qz = sy*cp*cr - cy*sp*sr;

q = [qw; qx; qy; qz];

% Normalize for safety
qnorm = sqrt(qw*qw + qx*qx + qy*qy + qz*qz);
if qnorm > 1e-12
    q = q / qnorm;
else
    q = [1; 0; 0; 0];
end

end


function c = cross3(a, b)
% cross3
%
% Manual 3D cross product for code generation clarity.

c = [ ...
    a(2)*b(3) - a(3)*b(2);
    a(3)*b(1) - a(1)*b(3);
    a(1)*b(2) - a(2)*b(1) ];

end

== matlab function Pretty_Lin_Hover_Sim/State Estimation/My Accel LPF ==
  data: x input; xlpf output; accel_alpha input
function xlpf = lpf(x, accel_alpha)

persistent prevx_accel firstrun_accel

if isempty(firstrun_accel)
    prevx_accel = x;
    firstrun_accel = 1;
end

xlpf = (1-accel_alpha)*prevx_accel + accel_alpha*x;

prevx_accel = xlpf;

end

== matlab function Pretty_Lin_Hover_Sim/State Estimation/My Gyro LPF ==
  data: x input; xlpf output; gyro_alpha input
function xlpf = lpf(x,gyro_alpha)

persistent prevx_gyro firstrun_gyro

if isempty(firstrun_gyro)
    prevx_gyro = x;
    firstrun_gyro = 1;
end

xlpf = (1-gyro_alpha)*prevx_gyro + gyro_alpha*x;

prevx_gyro = xlpf;

end
